simulink model "verify_Combustion_Calculation_mdl"  (R2016b)
settings: Solver=VariableStepDiscrete  StartTime=0.0  StopTime=1  MaxStep=1  RelTol=1e-3  EnableMultiTasking=on
libraries: carnot x2
settings Model: Creator=drhf  LastModifiedBy=srrt
settings DataIOCC: LimitDataPoints=on  SaveFormat=Array  SignalLoggingSaveFormat=ModelDataLogs
settings OptimizationCC: ExpressionDepthLimit=2147483647  LifeSpan=inf
settings DebuggingCC: UnderspecifiedInitializationDetection=Classic  MergeDetectMultiDrivingBlocksExec=none  SolverPrmCheckMsg=warning  FcnCallInpInsideContextMsg=warning  StateNameClashWarn=warning  SFUnexpectedBacktrackingDiag=warning  SFNoUnconditionalDefaultTransitionDiag=warning  SFExecutionAtInitializationDiag=none
settings HardwareCC: ProdBitPerPointer=32  ProdBitPerSizeT=32  ProdBitPerPtrDiffT=32  ProdLargestAtomicFloat=None  ProdIntDivRoundTo=Undefined  ProdEndianess=Unspecified  ProdWordSize=32  ProdHWDeviceType=32-bit Generic
settings ModelReferenceCC: PropagateSignalLabelsOutOfModel=off
settings GRTTargetCC: TargetLangStandard=C89/C90 (ANSI)  GeneratePreprocessorConditionals=Disable all  CombineOutputUpdateFcns=off  GRTInterface=on
settings ConfigComp: CovMetricSettings=dw  CovHtmlReporting=on  CovSaveCumulativeToWorkspaceVar=on  CovSaveSingleToWorkspaceVar=on  CovExternalEMLEnable=off

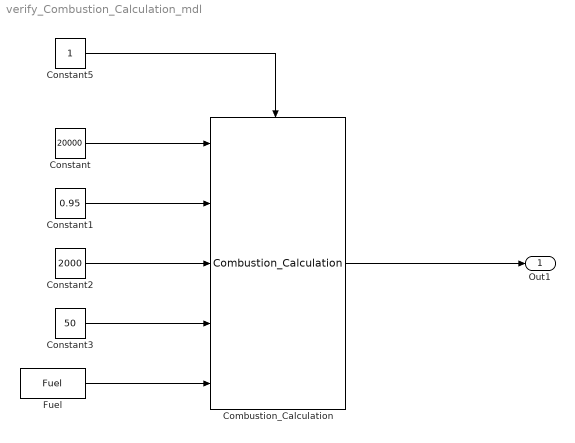
== system verify_Combustion_Calculation_mdl ==
  Combustion_Calculation : carnot/Basic/Thermal_Models/Combustion_Calculation
  Constant : Constant  Value=20000
  Constant1 : Constant  Value=0.95
  Constant2 : Constant  Value=2000
  Constant3 : Constant  Value=50
  Constant5 : Constant
  Fuel : carnot/Source/Energy/Fuel  ft=1  t=20  ls=3.5  p=1.013e5  h_values=[5.14e7 5.69e7]  tc=45  price=1  mass=[0.33 0.67 0 0 0 0]
  Out1 : Outport
  wires:
  Combustion_Calculation/1 -> Out1/1
  Constant5/1 -> Combustion_Calculation/Enable
  Constant2/1 -> Combustion_Calculation/3
  Constant3/1 -> Combustion_Calculation/4
  Fuel/1 -> Combustion_Calculation/5
  Constant/1 -> Combustion_Calculation/1
  Constant1/1 -> Combustion_Calculation/2
